simulink model "Motor4_Avellaneda"  (R2023b)
settings: Solver=VariableStepAuto  StartTime=0.0  StopTime=10  RelTol=1e-3
undefined symbols (not defined in the file or in its folder): A, B, C, Fc, K, K_I, L
settings Model: Creator=Usuario  LastModifiedBy=Usuario

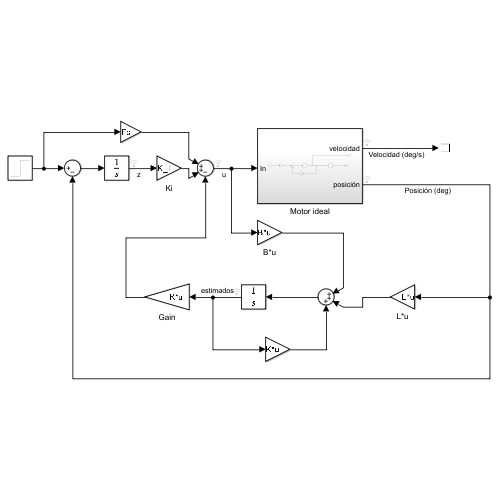
[thumbnail: Simulink's stored preview of the top-level diagram]
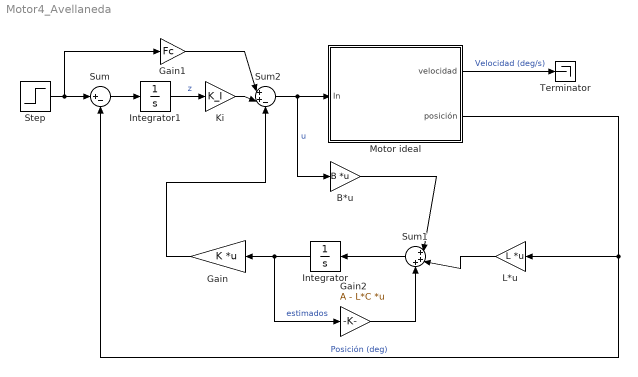
== system Motor4_Avellaneda ==
  B*u : Gain  Gain=B  Multiplication=Matrix(K*u)
  Gain : Gain  Gain=K  Multiplication=Matrix(K*u)
  Gain1 : Gain  Gain=Fc
  Gain2 : Gain  Gain=A - L*C  Multiplication=Matrix(K*u)
  Integrator : Integrator
  Integrator1 : Integrator
  Ki : Gain  Gain=K_I
  L*u : Gain  Gain=L  Multiplication=Matrix(K*u)
  Motor ideal : Subsystem
  Step : Step  Time=0  After=720  SampleTime=0
  Sum : Sum  Inputs=|+-
  Sum1 : Sum  Inputs=|+++
  Sum2 : Sum  Inputs=|++-
  Terminator : Terminator
  wires:
  Motor ideal/1(velocidad) -> Terminator/1  "Velocidad (deg/s)"
  Motor ideal/2(posición) -> Sum/2, L*u/1  "Posición (deg)"
  B*u/1 -> Sum1/1
  L*u/1 -> Sum1/2
  Sum1/1 -> Integrator/1
  Integrator/1 -> Gain2/1, Gain/1  "estimados"
  Gain2/1 -> Sum1/3
  Step/1 -> Gain1/1, Sum/1
  Sum/1 -> Integrator1/1
  Integrator1/1 -> Ki/1  "z"
  Sum2/1 -> B*u/1, Motor ideal/1(In)  "u"
  Ki/1 -> Sum2/2
  Gain1/1 -> Sum2/1
  Gain/1 -> Sum2/3

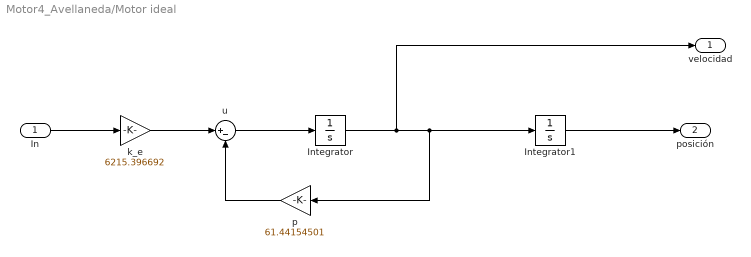
== system Motor4_Avellaneda/Motor ideal ==
  In : Inport
  Integrator : Integrator  InitialCondition=1
  Integrator1 : Integrator  InitialCondition=2
  k_e : Gain  Gain=6215.396692
  p : Gain  Gain=61.44154501
  u : Sum  Inputs=|+-
  velocidad : Outport
  posición : Outport  Port=2
  wires:
  Integrator/1 -> Integrator1/1, p/1, velocidad/1
  u/1 -> Integrator/1
  p/1 -> u/2
  k_e/1 -> u/1
  Integrator1/1 -> posición/1
  In/1 -> k_e/1
